simulink model "Band_pass"  (R2018a)
settings: Solver=VariableStepAuto  StartTime=0.0  StopTime=0.1  RelTol=1e-3
libraries: dsparch4 x1
settings Model: Creator=AlexZ  LastModifiedBy=AlexZ

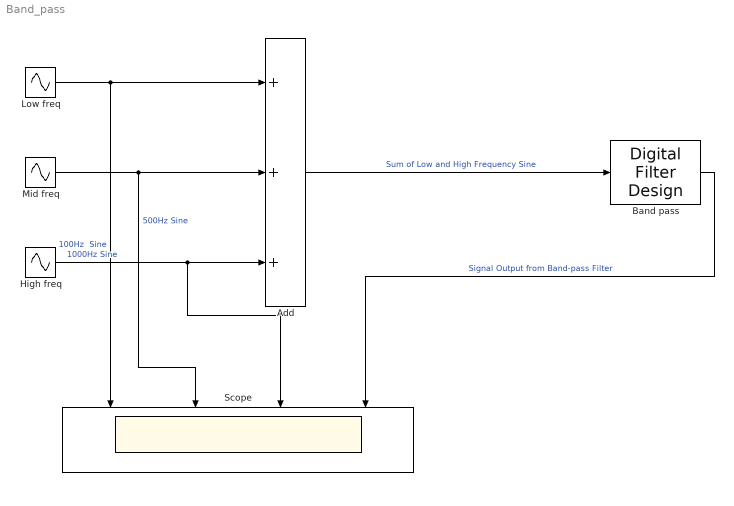
== system Band_pass ==
  Add : Sum  Inputs=+++
  "Band pass " : dsparch4/Digital Filter Design  mwdsp_browser_bugfix_var=off
  "High freq " : Sin  Frequency=2*pi*1000  Samples=1000  SampleTime=1e-5
  "Low freq " : Sin  Frequency=2*pi*100  SampleTime=1e-5
  Mid freq : Sin  Frequency=2*pi*500  SampleTime=1e-5  VectorParams1D=off
  Scope : Scope  NumInputPorts=4
  wires:
  "Low freq "/1 -> Add/1, Scope/1  "100Hz  Sine"
  "Band pass "/1 -> Scope/4  "Signal Output from Band-pass Filter"
  "High freq "/1 -> Scope/3, Add/3  "1000Hz Sine"
  Add/1 -> "Band pass "/1  "Sum of Low and High Frequency Sine"
  Mid freq/1 -> Scope/2, Add/2  "500Hz Sine"
